simulink model "pendule_inv_echant_etu"  (R2021a)
settings: Solver=VariableStepAuto  StartTime=0.0  StopTime=10.0  RelTol=1e-3
values from neighbouring files (symbols this model uses):
  delta_t = 0.4    [simu_pendule_inv_echant_etu.m]
  K = [10 1]    [simu_pendule_inv_capteur_etu.m]    (also in simu_pendule_inv_echant_etu.m = [30 10]; simu_pendule_inv_etu.m = [30 10])
  ue = 0    [simu_pendule_inv_capteur_etu.m]    (also in simu_pendule_inv_echant_etu.m; simu_pendule_inv_etu.m)
  x0 = [pi/20 0]'    [simu_pendule_inv_capteur_etu.m]    (also in simu_pendule_inv_echant_etu.m; simu_pendule_inv_etu.m = [pi/10 0]')
  xe = [0 0]'    [simu_pendule_inv_capteur_etu.m]    (also in simu_pendule_inv_echant_etu.m; simu_pendule_inv_etu.m)
undefined symbols (not defined in the file or in its folder): DiscIntNeverNeededParam
settings Model: Creator=abennagh  LastModifiedBy=abennagh

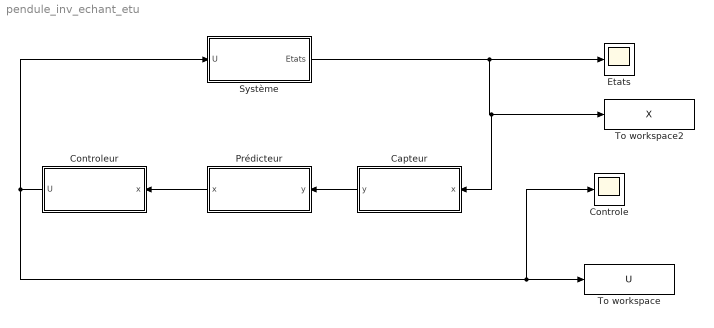
== system pendule_inv_echant_etu ==
  Capteur : Subsystem
  Controle : Scope
  Controleur : Subsystem
  Etats : Scope
  Prédicteur : Subsystem
  Système : Subsystem
  To workspace : ToWorkspace  VariableName=U  SaveFormat=Timeseries  SampleTime=-1
  To workspace2 : ToWorkspace  VariableName=X  SaveFormat=Timeseries  SampleTime=-1
  wires:
  Système/1(Etats) -> Capteur/1(x), To workspace2/1, Etats/1
  Prédicteur/1(x) -> Controleur/1(x)
  Controleur/1(U) -> Controle/1, To workspace/1, Système/1(U)
  Capteur/1(y) -> Prédicteur/1(y)

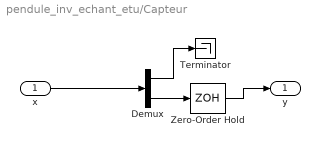
== system pendule_inv_echant_etu/Capteur ==
  x : Inport
  Demux : Demux  Outputs=2
  Terminator : Terminator
  Zero-Order Hold : ZeroOrderHold  SampleTime=delta_t
  y : Outport
  wires:
  Demux/1 -> Terminator/1
  Demux/2 -> Zero-Order Hold/1
  Zero-Order Hold/1 -> y/1
  x/1 -> Demux/1

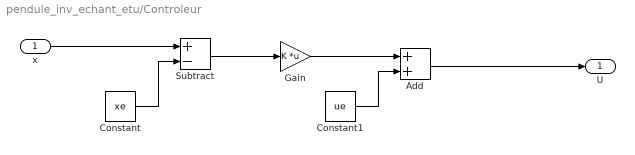
== system pendule_inv_echant_etu/Controleur ==
  x : Inport
  Add : Sum
  Constant : Constant  Value=xe
  Constant1 : Constant  Value=ue
  Gain : Gain  Gain=K  Multiplication=Matrix(K*u)
  Subtract : Sum  Inputs=+-
  U : Outport
  wires:
  x/1 -> Subtract/1
  Constant/1 -> Subtract/2
  Subtract/1 -> Gain/1
  Add/1 -> U/1
  Gain/1 -> Add/1
  Constant1/1 -> Add/2

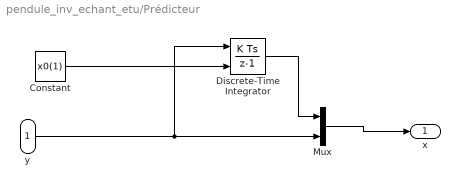
== system pendule_inv_echant_etu/Prédicteur ==
  y : Inport
  Constant : Constant  Value=x0(1)  OutDataTypeStr=double
  Discrete-Time Integrator : DiscreteIntegrator  InitialConditionSource=external  SampleTime=-1  ICPrevOutput=DiscIntNeverNeededParam  ICPrevScaledInput=DiscIntNeverNeededParam
  Mux : Mux  Inputs=2
  x : Outport
  wires:
  y/1 -> Discrete-Time Integrator/1, Mux/2
  Mux/1 -> x/1
  Constant/1 -> Discrete-Time Integrator/2
  Discrete-Time Integrator/1 -> Mux/1

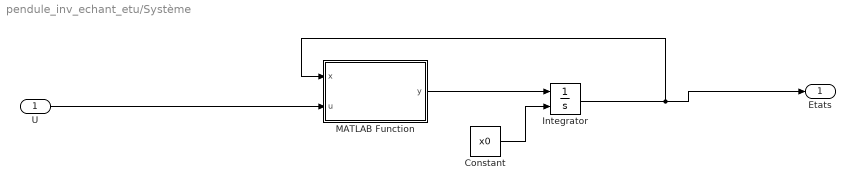
== system pendule_inv_echant_etu/Système ==
  U : Inport
  Constant : Constant  Value=x0
  Integrator : Integrator  InitialConditionSource=external
  MATLAB Function : MATLAB Function  TreatAsAtomicUnit=on
  Etats : Outport
  wires:
  U/1 -> MATLAB Function/2(u)
  MATLAB Function/1(y) -> Integrator/1
  Integrator/1 -> MATLAB Function/1(x), Etats/1
  Constant/1 -> Integrator/2

== matlab function pendule_inv_echant_etu/Système/MATLAB Function ==
  data: x input; u input; y output
function y = fcn(x,u)
g = 9.81; l = 10;   % constantes
y = [x(2); (g/l)*sin(x(1))-(cos(x(1))*u)/l];
